simulink model "emo_1wr8_task"  (Simulink 3.00)
libraries: logiclib x5, genlib x4, mathlib x3, analoglib x2, execlib x1, inoutlib x1

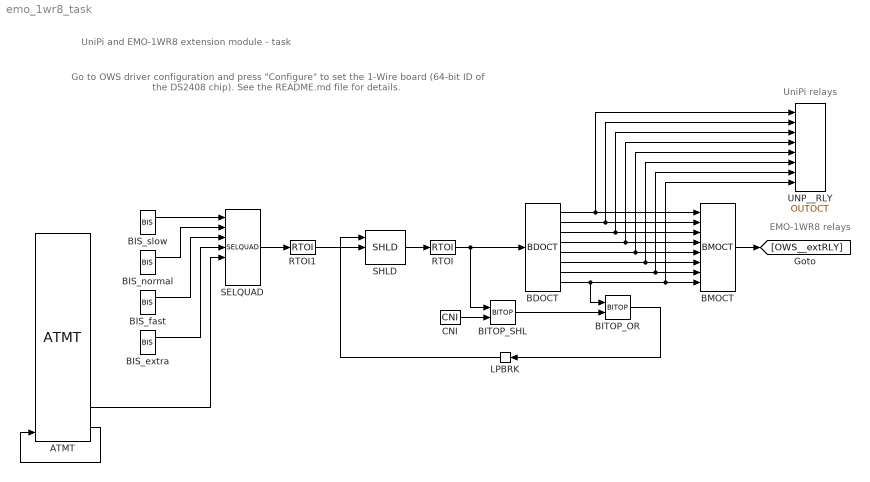
== system emo_1wr8_task ==
  note: UniPi relays
  note: EMO-1WR8 relays
  note: Go to OWS driver configuration and press "Configure" to set the 1-Wire board (64-bit ID of the DS2408 chip).
      |
      | See the README.md file for details.
  note: UniPi and EMO-1WR8 extension module - task
  ATMT : logiclib/ATMT  morestps=off  ntr=4  STT=[0 15 1; 1 15 2; 2 15 3; 3 15 0]  touts=[5.6 2.4 2.4 2.4 5 6 7 8 9 10 11 12 13 14 15 16]
  BDOCT : logiclib/BDOCT  shift=0
  BIS_extra : genlib/BIS  Y0=off  t1=0.05  t2=0.1  t3=0  t4=4  t5=5  t6=6  t7=7  t8=8  RPT=on
  BIS_fast : genlib/BIS  Y0=off  t1=0.1  t2=0.2  t3=0  t4=4  t5=5  t6=6  t7=7  t8=8  RPT=on
  BIS_normal : genlib/BIS  Y0=off  t1=0.2  t2=0.4  t3=0  t4=4  t5=5  t6=6  t7=7  t8=8  RPT=on
  BIS_slow : genlib/BIS  Y0=off  t1=0.4  t2=0.8  t3=0  t4=4  t5=5  t6=6  t7=7  t8=8  RPT=on
  BITOP_OR : logiclib/BITOP  iop=2: Bit OR
  BITOP_SHL : logiclib/BITOP  iop=5: Shift Left
  BMOCT : logiclib/BMOCT  shift=0
  CNI : mathlib/CNI  icn=1
  LPBRK : execlib/LPBRK  Orientation=left
  RTOI : mathlib/RTOI
  RTOI1 : mathlib/RTOI
  SELQUAD : analoglib/SELQUAD  BINF=off
  SHLD : analoglib/SHLD  y0=7  mode=1: Triggered sampling
  UNP__RLY : inoutlib/OUTOCT
  wires:
  ATMT/17 -> SELQUAD/5
  ATMT/19 -> ATMT/20
  BDOCT/1 -> BMOCT/1, UNP__RLY/1
  BDOCT/2 -> BMOCT/2, UNP__RLY/2
  BDOCT/3 -> BMOCT/3, UNP__RLY/3
  BDOCT/4 -> BMOCT/4, UNP__RLY/4
  BDOCT/5 -> BMOCT/5, UNP__RLY/5
  BDOCT/6 -> BMOCT/6, UNP__RLY/6
  BDOCT/7 -> BMOCT/7, UNP__RLY/7
  BDOCT/8 -> BITOP_OR/1, BMOCT/8, UNP__RLY/8
  BIS_extra/1 -> SELQUAD/4
  BIS_fast/1 -> SELQUAD/3
  BIS_normal/1 -> SELQUAD/2
  BIS_slow/1 -> SELQUAD/1
  BITOP_OR/1 -> LPBRK/1
  BITOP_SHL/1 -> BITOP_OR/2
  BMOCT/1 -> [OWS__extRLY]
  CNI/1 -> BITOP_SHL/2
  LPBRK/1 -> SHLD/1
  RTOI/1 -> BDOCT/1, BITOP_SHL/1
  RTOI1/1 -> SHLD/2
  SELQUAD/1 -> RTOI1/1
  SHLD/1 -> RTOI/1
